simulink model "torch_arm_telem"  (R2024a)
settings: Solver=FixedStepAuto  StartTime=0.0  StopTime=50  FixedStep=framePeriod_s  RelTol=1e-3
undefined symbols (not defined in the file): Aircraft, DiscIntNeverNeededParam, framePeriod_s, frameRate_hz, magnitude
libraries: simulink x42, slpidlib x13, dspmathops x1, simulink_extras x1
(part 2 of 4)

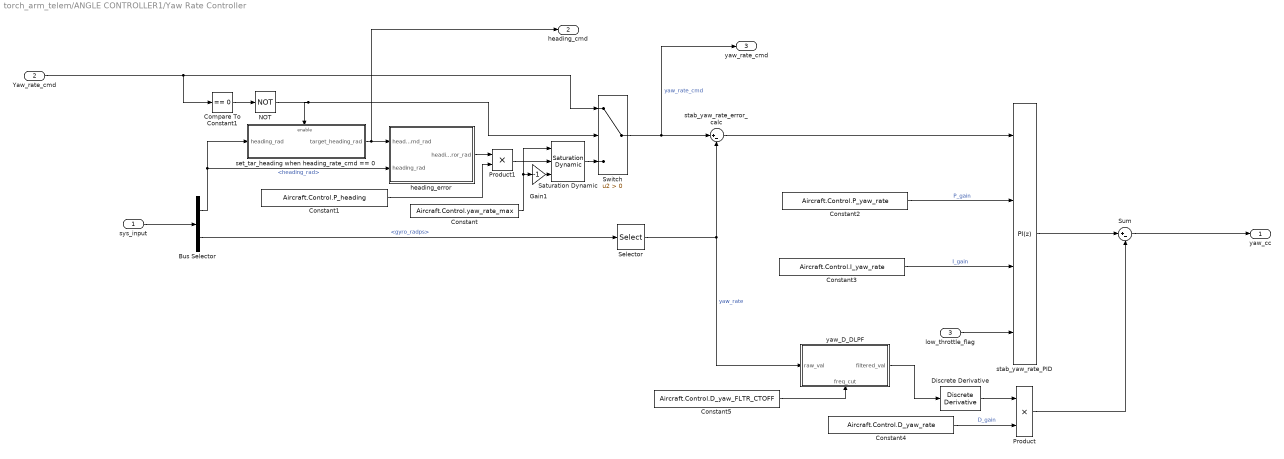
== system torch_arm_telem/ANGLE CONTROLLER1/Yaw Rate Controller ==
  sys_input : Inport
  Yaw_rate_cmd : Inport  Port=2
  low_throttle_flag : Inport  Port=3
  Bus Selector : BusSelector  OutputSignals=StateEstData.bfs_ins.heading_rad,StateEstData.bfs_ins.gyro_radps
  Compare To Constant1 : simulink/Logic and Bit Operations/Compare To Constant  relop===  const=0  OutDataTypeStr=boolean
  Constant : Constant  Value=Aircraft.Control.yaw_rate_max
  Constant1 : Constant  Value=Aircraft.Control.P_heading  OutDataTypeStr=single
  Constant2 : Constant  Value=Aircraft.Control.P_yaw_rate  OutDataTypeStr=single
  Constant3 : Constant  Value=Aircraft.Control.I_yaw_rate  OutDataTypeStr=single
  Constant4 : Constant  Value=Aircraft.Control.D_yaw_rate  OutDataTypeStr=single
  Constant5 : Constant  Value=Aircraft.Control.D_yaw_FLTR_CTOFF  OutDataTypeStr=single
  Discrete Derivative : simulink/Quick Insert/Discrete/Discrete Derivative  gainval=1.0  ICPrevScaledInput=0.0  OutMin=[]  OutMax=[]  OutDataType=fixdt(1, 16)  OutScaling=2^-10  DoSatur=off
  Gain1 : Gain  Gain=-1
  NOT : Logic  Operator=NOT  IconShape=distinctive  AllPortsSameDT=off  OutDataTypeStr=boolean
  Product : Product
  Product1 : Product
  Saturation Dynamic : simulink/Discontinuities/Saturation Dynamic  OutMin=[]  OutMax=[]  OutDataTypeStr=Inherit: Same as second input  OutDataType=fixdt(1, 16)  OutScaling=2^-10  DoSatur=off
  Selector : Selector  InputPortWidth=3  IndexOptions=Index vector (dialog)  Indices=3  OutputSizes=1
  Sum : Sum  Inputs=|+-
  Switch : Switch  Criteria=u2 > Threshold  SaturateOnIntegerOverflow=off  InputSameDT=off
  heading_error : Subsystem
  set_tar_heading when heading_rate_cmd == 0 : Subsystem  TreatAsAtomicUnit=on
  stab_yaw_rate_PID : slpidlib/PID Controller  Controller=PI  Form=Parallel  TimeDomain=Discrete-time  UseExternalTs=off  SampleTime=framePeriod_s  IntegratorMethod=Forward Euler  FilterMethod=Forward Euler  ControllerParametersSource=external  P=1.85  I=0.01  UseKiTs=off  D=0  UseExternalDerivativeSource=off  N=100  UseFilter=off  TunerSelectOption=Transfer Function Based (PID Tuner App)  InitialConditionSource=internal  InitialConditionForIntegrator=0  InitialConditionForFilter=0  DifferentiatorICPrevScaledInput=0  ExternalReset=either  TrackingMode=off  Kt=1  LimitOutput=on  SatLimitsSource=internal  UpperSaturationLimit=1  LowerSaturationLimit=-1  LinearizeAsGain=off  AntiWindupMode=clamping  Kb=1  LimitIntegrator=off  UpperIntegratorSaturationLimit=inf  LowerIntegratorSaturationLimit=-inf  POutMin=[]  POutMax=[]  IOutMin=[]  IOutMax=[]  DOutMin=[]  DOutMax=[]  NOutMin=[]  NOutMax=[]  SumOutMin=[]  SumOutMax=[]  SaturationOutMin=[]  SaturationOutMax=[]  PParamMin=[]  PParamMax=[]  IParamMin=[]  IParamMax=[]  DParamMin=[]  DParamMax=[]  NParamMin=[]  NParamMax=[]  KbParamMin=[]  KbParamMax=[]  KtParamMin=[]  KtParamMax=[]  KbOutMin=[]  KbOutMax=[]  KtOutMin=[]  KtOutMax=[]  IntegratorOutMin=[]  IntegratorOutMax=[]  FilterOutMin=[]  FilterOutMax=[]  SumI1OutMin=[]  SumI1OutMax=[]  SumI2OutMin=[]  SumI2OutMax=[]  SumI3OutMin=[]  SumI3OutMax=[]  SumI4OutMin=[]  SumI4OutMax=[]  SumDOutMin=[]  SumDOutMax=[]  DifferentiatorOutMin=[]  DifferentiatorOutMax=[]  FilterDiffOutCoefMin=[]  FilterDiffOutCoefMax=[]  ReciprocalOutMin=[]  ReciprocalOutMax=[]  SumDenOutMin=[]  SumDenOutMax=[]  SumNumOutMin=[]  SumNumOutMax=[]  DivideOutMin=[]  DivideOutMax=[]  UdiffTsProdOutMin=[]  UdiffTsProdOutMax=[]  NTsProdOutMin=[]  NTsProdOutMax=[]  UintegralTsProdOutMin=[]  UintegralTsProdOutMax=[]  UngainTsProdOutMin=[]  UngainTsProdOutMax=[]  ClampingZeroOutDataTypeStr=Inherit: Inherit via back propagation  ClampingZeroOutMin=[]  ClampingZeroOutMax=[]  FilterDenConstantOutDataTypeStr=Inherit: Inherit via back propagation  FilterDenConstantOutMin=[]  FilterDenConstantOutMax=[]  PCopyOutDataTypeStr=Inherit: Inherit via back propagation  PCopyOutMin=[]  PCopyOutMax=[]  NCopyOutDataTypeStr=Inherit: Inherit via back propagation  NCopyOutMin=[]  NCopyOutMax=[]  IntegratorContinuousStateAttributes=''  IntegratorStateMustResolveToSignalObject=off  IntegratorRTWStateStorageClass=Auto  FilterContinuousStateAttributes=''  FilterStateMustResolveToSignalObject=off  FilterRTWStateStorageClass=Auto  ParallelPVariant=ExternalParameters  IdealPVariant=Disabled  IVariant=ExternalParameters  DVariant=Disabled  IntegratorVariant=Discrete  SatVariant=Enabled  AWVariant=DiscClampingParallel  PCopyVariant=Disabled  TRVariant=Disabled  FdbkBlocksVariant=Forward  IdealPFdbkVariant=Disabled  SatFdbkVariant=Disabled  DerivativeFilterVariant=Disabled  NVariant=Disabled  NCopyVariant=Disabled_SignalSpec  FilterICVariant=Disabled  IntegratorICVariant=InternalICs  ExternalResetVariant=ExternalReset  TRSumVariant=Passthrough  SumFdbkVariant=Disabled  SumVariant=Sum_PI  TsampFilterVariant=InternalTs  TsampNgainVariant=Passthrough  TsampIntegralVariant=Disabled_SignalSpec  ExternalSaturationOutDataTypeStr=Inherit: Same as second input  DerivativeSourceVariant=Disabled
  stab_yaw_rate_error_calc : Sum  Inputs=|+-
  yaw_D_DLPF : Subsystem
      settings: PortSchema="{\"entries\":[{\"content\":{\"sides\":[{\"content\":{\"connectorIds\":[\"In1\"]},\"type\":\"ConnectorPlacement.EquallySpacedRectSide\",\"uuid\":\"20236834-aeb3-4c5b-bb2e-f84447e752b5\"},{\"content\":{\"connectorIds\":[\"Out1\"],\"side\":\"RIGHT\"},\"type\":\"ConnectorPlacement.EquallySpacedRectSide\",\"uuid\":\"d668f9a1-a3df-4207-8bf1-99fb838e59b2\"},{\"content\":{\"connectorIds\":[],\"side\":\"TOP\"},\"type\":\"ConnectorPlacement.EquallySpacedRectSide\",\"uuid\":\"66cceb06-f4bc-4278-b965-2427292e46df\"},{\"content\":{\"connectorIds\":[\"In2\"],\"side\":\"BOTTOM\"},\"type\":\"ConnectorPlacement.EquallySpacedRectSide\",\"uuid\":\"8fdaac6a-cb03-4bd4-87bb-7bafd10bc297\"}]},\"type\":\"ConnectorPlacement.EquallySpacedConnector\",\"uuid\":\"3dc29a9a-e794-478d-b7df-452e6c2d3f66\"}],\"packageUris\":[\"http://schema.mathworks.com/mf0/Connector/R2020b\"],\"version\":\"1.0\"}"
  yaw_cc : Outport
  heading_cmd : Outport  Port=2
  yaw_rate_cmd : Outport  Port=3
  wires:
  sys_input/1 -> Bus Selector/1
  Bus Selector/2 -> Selector/1  "<gyro_radps>"
  stab_yaw_rate_PID/1 -> Sum/1
  Sum/1 -> yaw_cc/1
  Product/1 -> Sum/2
  Discrete Derivative/1 -> Product/1
  Constant2/1 -> stab_yaw_rate_PID/2  "P_gain"
  Constant3/1 -> stab_yaw_rate_PID/3  "I_gain"
  Constant4/1 -> Product/2  "D_gain"
  Selector/1 -> stab_yaw_rate_error_calc/2, yaw_D_DLPF/1(raw_val)  "yaw_rate"
  low_throttle_flag/1 -> stab_yaw_rate_PID/4
  Compare To Constant1/1 -> NOT/1
  Bus Selector/1 -> set_tar_heading when heading_rate_cmd == 0/1(heading_rad), heading_error/2(heading_rad)  "<heading_rad>"
  Switch/1 -> yaw_rate_cmd/1, stab_yaw_rate_error_calc/1  "yaw_rate_cmd"
  Yaw_rate_cmd/1 -> Switch/1, Compare To Constant1/1
  heading_error/1(heading_error_rad) -> Product1/1
  Constant1/1 -> Product1/2
  NOT/1 -> Switch/2, set_tar_heading when heading_rate_cmd == 0/Enable
  set_tar_heading when heading_rate_cmd == 0/1(target_heading_rad) -> heading_cmd/1, heading_error/1(heading_cmd_rad)
  Product1/1 -> Saturation Dynamic/2
  Saturation Dynamic/1 -> Switch/3
  Gain1/1 -> Saturation Dynamic/3
  Constant/1 -> Saturation Dynamic/1, Gain1/1
  Constant5/1 -> yaw_D_DLPF/2(freq_cut)
  yaw_D_DLPF/1(filtered_val) -> Discrete Derivative/1
  stab_yaw_rate_error_calc/1 -> stab_yaw_rate_PID/1

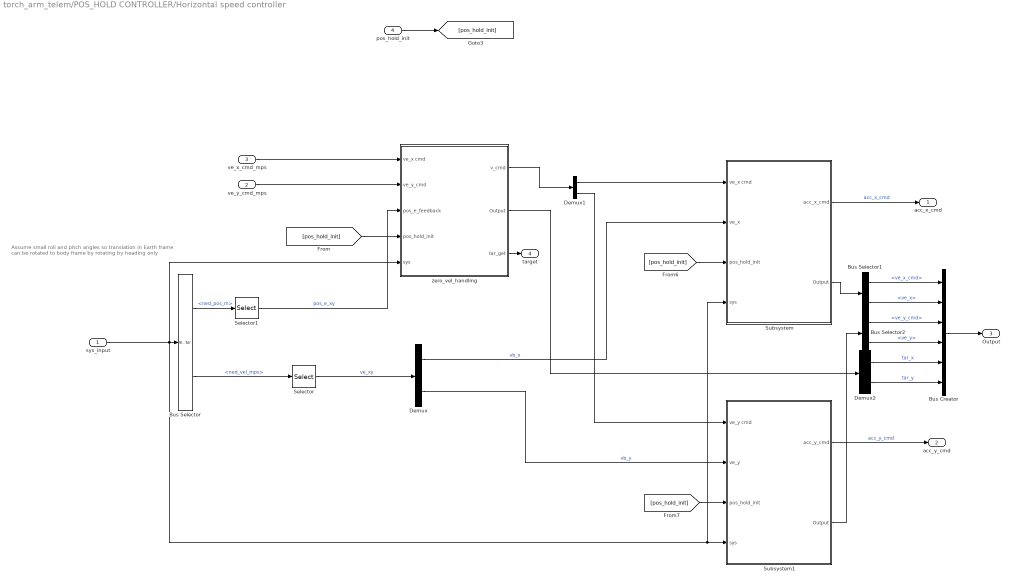
== system torch_arm_telem/POS_HOLD CONTROLLER/Horizontal speed controller ==
  note: Assume small roll and pitch angles so translation in Earth frame can be rotated to body frame by rotating by heading only
  sys_input : Inport
  ve_y_cmd_mps : Inport  Port=2
  ve_x_cmd_mps : Inport  Port=3
  pos_hold_init : Inport  Port=4
  Bus Creator : BusCreator  Inputs=6
  Bus Selector : BusSelector  OutputSignals=StateEstData.aux_ins.ned_pos_m,StateEstData.bfs_ins.ned_vel_mps
  Bus Selector1 : BusSelector  OutputSignals=ve_x_cmd,ve_x
  Bus Selector2 : BusSelector  OutputSignals=ve_y_cmd,ve_y
  Demux : Demux  Outputs=2
  Demux1 : Demux  Outputs=2
  Demux2 : Demux  Outputs=2
  Selector : Selector  InputPortWidth=3  IndexOptions=Index vector (dialog)  Indices=[1 2]  OutputSizes=1
  Selector1 : Selector  InputPortWidth=3  IndexOptions=Index vector (dialog)  Indices=[1 2]  OutputSizes=1
  Subsystem : Subsystem
  Subsystem1 : Subsystem
  zero_vel_handling : Subsystem
  acc_x_cmd : Outport
  acc_y_cmd : Outport  Port=2
  Output : Outport  Port=3
  target : Outport  Port=4
  wires:
  Subsystem1/1(acc_y_cmd) -> acc_y_cmd/1  "acc_y_cmd"
  Subsystem/1(acc_x_cmd) -> acc_x_cmd/1  "acc_x_cmd"
  sys_input/1 -> Bus Selector/1, Subsystem/4(sys), Subsystem1/4(sys), zero_vel_handling/5(sys)
  Bus Selector/2 -> Selector/1  "<ned_vel_mps>"
  Demux/1 -> Subsystem/2(ve_x)  "vb_x"
  pos_hold_init/1 -> [pos_hold_init]
  [pos_hold_init] -> Subsystem/3(pos_hold_init)
  [pos_hold_init] -> Subsystem1/3(pos_hold_init)
  Subsystem/2(Output) -> Bus Selector1/1
  Subsystem1/2(Output) -> Bus Selector2/1
  Bus Selector1/1 -> Bus Creator/1  "<ve_x_cmd>"
  Bus Selector1/2 -> Bus Creator/2  "<ve_x>"
  Bus Selector2/1 -> Bus Creator/3  "<ve_y_cmd>"
  Bus Selector2/2 -> Bus Creator/4  "<ve_y>"
  Bus Creator/1 -> Output/1
  Bus Selector/1 -> Selector1/1  "<ned_pos_m>"
  Demux/2 -> Subsystem1/2(ve_y)  "vb_y"
  ve_x_cmd_mps/1 -> zero_vel_handling/1(ve_x cmd)
  ve_y_cmd_mps/1 -> zero_vel_handling/2(ve_y_cmd)
  Selector1/1 -> zero_vel_handling/3(pos_e_feedback)  "pos_e_xy"
  [pos_hold_init] -> zero_vel_handling/4(pos_hold_init)
  zero_vel_handling/1(v_cmd) -> Demux1/1
  Demux1/1 -> Subsystem/1(ve_x cmd)
  Demux1/2 -> Subsystem1/1(ve_y cmd)
  zero_vel_handling/2(Output) -> Demux2/1
  Demux2/1 -> Bus Creator/5  "tar_x"
  Demux2/2 -> Bus Creator/6  "tar_y"
  Selector/1 -> Demux/1  "ve_xy"
  zero_vel_handling/3(tar_get) -> target/1

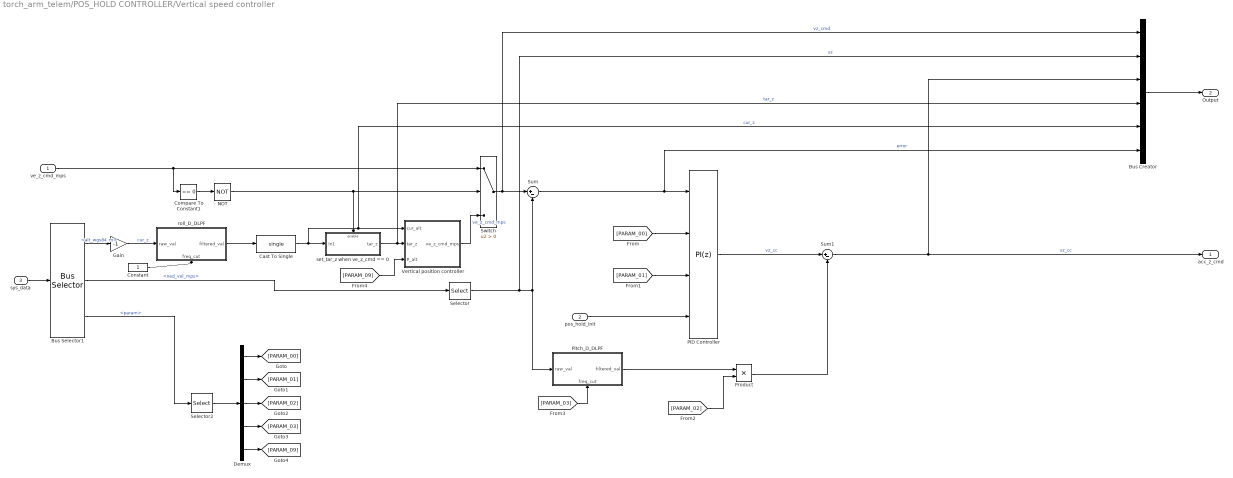
== system torch_arm_telem/POS_HOLD CONTROLLER/Vertical speed controller ==
  ve_z_cmd_mps : Inport
  pos_hold_init : Inport  Port=2
  sys_data : Inport  Port=3
  Bus Creator : BusCreator  Inputs=6
  Bus Selector1 : BusSelector  OutputSignals=Sensor Data.ext_gnss1.alt_wgs84_m,StateEstData.bfs_ins.ned_vel_mps,Telemetry Data.param
  Cast To Single : DataTypeConversion  OutDataTypeStr=single  SaturateOnIntegerOverflow=off  RndMeth=Floor
  Compare To Constant1 : simulink/Logic and Bit Operations/Compare To Constant  relop===  const=0  OutDataTypeStr=boolean
  Constant : Constant  OutDataTypeStr=single
  Demux : Demux  Outputs=5
  Gain : Gain  Gain=-1
  NOT : Logic  Operator=NOT  IconShape=distinctive  AllPortsSameDT=off  OutDataTypeStr=boolean
  PID Controller : slpidlib/PID Controller  Controller=PI  Form=Parallel  TimeDomain=Discrete-time  UseExternalTs=off  SampleTime=framePeriod_s  IntegratorMethod=Forward Euler  FilterMethod=Forward Euler  ControllerParametersSource=external  P=0  I=0  UseKiTs=off  D=0  UseExternalDerivativeSource=off  N=100  UseFilter=off  TunerSelectOption=Frequency Response Based  InitialConditionSource=internal  InitialConditionForIntegrator=0  InitialConditionForFilter=0  DifferentiatorICPrevScaledInput=0  ExternalReset=either  TrackingMode=off  Kt=1  LimitOutput=on  SatLimitsSource=internal  UpperSaturationLimit=1  LowerSaturationLimit=-1  LinearizeAsGain=on  AntiWindupMode=clamping  Kb=1  LimitIntegrator=off  UpperIntegratorSaturationLimit=inf  LowerIntegratorSaturationLimit=-inf  POutMin=[]  POutMax=[]  IOutMin=[]  IOutMax=[]  DOutMin=[]  DOutMax=[]  NOutMin=[]  NOutMax=[]  SumOutMin=[]  SumOutMax=[]  SaturationOutMin=[]  SaturationOutMax=[]  PParamMin=[]  PParamMax=[]  IParamMin=[]  IParamMax=[]  DParamMin=[]  DParamMax=[]  NParamMin=[]  NParamMax=[]  KbParamMin=[]  KbParamMax=[]  KtParamMin=[]  KtParamMax=[]  KbOutMin=[]  KbOutMax=[]  KtOutMin=[]  KtOutMax=[]  IntegratorOutMin=[]  IntegratorOutMax=[]  FilterOutMin=[]  FilterOutMax=[]  SumI1OutMin=[]  SumI1OutMax=[]  SumI2OutMin=[]  SumI2OutMax=[]  SumI3OutMin=[]  SumI3OutMax=[]  SumI4OutMin=[]  SumI4OutMax=[]  SumDOutMin=[]  SumDOutMax=[]  DifferentiatorOutMin=[]  DifferentiatorOutMax=[]  FilterDiffOutCoefMin=[]  FilterDiffOutCoefMax=[]  ReciprocalOutMin=[]  ReciprocalOutMax=[]  SumDenOutMin=[]  SumDenOutMax=[]  SumNumOutMin=[]  SumNumOutMax=[]  DivideOutMin=[]  DivideOutMax=[]  UdiffTsProdOutMin=[]  UdiffTsProdOutMax=[]  NTsProdOutMin=[]  NTsProdOutMax=[]  UintegralTsProdOutMin=[]  UintegralTsProdOutMax=[]  UngainTsProdOutMin=[]  UngainTsProdOutMax=[]  ClampingZeroOutDataTypeStr=Inherit: Inherit via back propagation  ClampingZeroOutMin=[]  ClampingZeroOutMax=[]  FilterDenConstantOutDataTypeStr=Inherit: Inherit via back propagation  FilterDenConstantOutMin=[]  FilterDenConstantOutMax=[]  PCopyOutDataTypeStr=Inherit: Inherit via back propagation  PCopyOutMin=[]  PCopyOutMax=[]  NCopyOutDataTypeStr=Inherit: Inherit via back propagation  NCopyOutMin=[]  NCopyOutMax=[]  IntegratorContinuousStateAttributes=''  IntegratorStateMustResolveToSignalObject=off  IntegratorRTWStateStorageClass=Auto  FilterContinuousStateAttributes=''  FilterStateMustResolveToSignalObject=off  FilterRTWStateStorageClass=Auto  ParallelPVariant=ExternalParameters  IdealPVariant=Disabled  IVariant=ExternalParameters  DVariant=Disabled  IntegratorVariant=Discrete  SatVariant=Enabled  AWVariant=DiscClampingParallel  PCopyVariant=Disabled  TRVariant=Disabled  FdbkBlocksVariant=Forward  IdealPFdbkVariant=Disabled  SatFdbkVariant=Disabled  DerivativeFilterVariant=Disabled  NVariant=Disabled  NCopyVariant=Disabled_SignalSpec  FilterICVariant=Disabled  IntegratorICVariant=InternalICs  ExternalResetVariant=ExternalReset  TRSumVariant=Passthrough  SumFdbkVariant=Disabled  SumVariant=Sum_PI  TsampFilterVariant=InternalTs  TsampNgainVariant=Passthrough  TsampIntegralVariant=Disabled_SignalSpec  ExternalSaturationOutDataTypeStr=Inherit: Same as second input  DerivativeSourceVariant=Disabled
  Pitch_D_DLPF : Subsystem
      settings: PortSchema="{\"entries\":[{\"content\":{\"sides\":[{\"content\":{\"connectorIds\":[\"In1\"]},\"type\":\"ConnectorPlacement.EquallySpacedRectSide\",\"uuid\":\"20236834-aeb3-4c5b-bb2e-f84447e752b5\"},{\"content\":{\"connectorIds\":[\"Out1\"],\"side\":\"RIGHT\"},\"type\":\"ConnectorPlacement.EquallySpacedRectSide\",\"uuid\":\"d668f9a1-a3df-4207-8bf1-99fb838e59b2\"},{\"content\":{\"connectorIds\":[],\"side\":\"TOP\"},\"type\":\"ConnectorPlacement.EquallySpacedRectSide\",\"uuid\":\"66cceb06-f4bc-4278-b965-2427292e46df\"},{\"content\":{\"connectorIds\":[\"In2\"],\"side\":\"BOTTOM\"},\"type\":\"ConnectorPlacement.EquallySpacedRectSide\",\"uuid\":\"7d08bc25-8e2d-44c6-8f94-b04e75c70268\"}]},\"type\":\"ConnectorPlacement.EquallySpacedConnector\",\"uuid\":\"3dc29a9a-e794-478d-b7df-452e6c2d3f66\"}],\"packageUris\":[\"http://schema.mathworks.com/mf0/Connector/R2020b\"],\"version\":\"1.0\"}"
  Product : Product
  Selector : Selector  InputPortWidth=3  IndexOptions=Index vector (dialog)  Indices=[3]  OutputSizes=1
  Selector2 : Selector  IndexMode=Zero-based  InputPortWidth=24  IndexOptions=Index vector (dialog)  Indices=[0 1 2 3 9]  OutputSizes=1
  Sum : Sum  Inputs=|+-
  Sum1 : Sum  Inputs=|+-
  Switch : Switch  Criteria=u2 > Threshold  SaturateOnIntegerOverflow=off  InputSameDT=off
  Vertical position controller : Subsystem
  roll_D_DLPF : Subsystem
      settings: PortSchema="{\"entries\":[{\"content\":{\"sides\":[{\"content\":{\"connectorIds\":[\"In1\"]},\"type\":\"ConnectorPlacement.EquallySpacedRectSide\",\"uuid\":\"20236834-aeb3-4c5b-bb2e-f84447e752b5\"},{\"content\":{\"connectorIds\":[\"Out1\"],\"side\":\"RIGHT\"},\"type\":\"ConnectorPlacement.EquallySpacedRectSide\",\"uuid\":\"d668f9a1-a3df-4207-8bf1-99fb838e59b2\"},{\"content\":{\"connectorIds\":[],\"side\":\"TOP\"},\"type\":\"ConnectorPlacement.EquallySpacedRectSide\",\"uuid\":\"66cceb06-f4bc-4278-b965-2427292e46df\"},{\"content\":{\"connectorIds\":[\"In2\"],\"side\":\"BOTTOM\"},\"type\":\"ConnectorPlacement.EquallySpacedRectSide\",\"uuid\":\"8fdaac6a-cb03-4bd4-87bb-7bafd10bc297\"}]},\"type\":\"ConnectorPlacement.EquallySpacedConnector\",\"uuid\":\"3dc29a9a-e794-478d-b7df-452e6c2d3f66\"}],\"packageUris\":[\"http://schema.mathworks.com/mf0/Connector/R2020b\"],\"version\":\"1.0\"}"
  set_tar_z when ve_z_cmd == 0 : Subsystem  TreatAsAtomicUnit=on
  acc_z_cmd : Outport
  Output : Outport  Port=2
  wires:
  [PARAM_00] -> PID Controller/2
  Bus Selector1/2 -> Selector/1  "<ned_vel_mps>"
  sys_data/1 -> Bus Selector1/1
  Pitch_D_DLPF/1(filtered_val) -> Product/1
  Selector/1 -> Bus Creator/2, Sum/2, Pitch_D_DLPF/1(raw_val)  "vz"
  [PARAM_02] -> Product/2
  Product/1 -> Sum1/2
  ve_z_cmd_mps/1 -> Compare To Constant1/1, Switch/1
  Compare To Constant1/1 -> NOT/1
  Switch/1 -> Bus Creator/1, Sum/1  "vz_cmd"
  set_tar_z when ve_z_cmd == 0/1(tar_z) -> Bus Creator/4, Vertical position controller/2(tar_z)  "tar_z"
  pos_hold_init/1 -> PID Controller/4
  [PARAM_03] -> Pitch_D_DLPF/2(freq_cut)
  [PARAM_09] -> Vertical position controller/3(P_alt)
  Bus Creator/1 -> Output/1
  Cast To Single/1 -> Bus Creator/5, Vertical position controller/1(cur_alt), set_tar_z when ve_z_cmd == 0/1(In1)  "cur_z"
  Sum/1 -> Bus Creator/6, PID Controller/1  "error"
  Sum1/1 -> acc_z_cmd/1, Bus Creator/3  "vz_cc"
  PID Controller/1 -> Sum1/1  "vz_cc"
  Bus Selector1/3 -> Selector2/1  "<param>"
  Selector2/1 -> Demux/1
  Demux/1 -> [PARAM_00]
  Demux/2 -> [PARAM_01]
  Demux/3 -> [PARAM_02]
  Demux/4 -> [PARAM_03]
  [PARAM_01] -> PID Controller/3
  Vertical position controller/1(ve_z_cmd_mps) -> Switch/3  "ve_z_cmd_mps"
  Demux/5 -> [PARAM_09]
  NOT/1 -> Switch/2, set_tar_z when ve_z_cmd == 0/Enable
  Bus Selector1/1 -> Gain/1  "<alt_wgs84_m>"
  Gain/1 -> roll_D_DLPF/1(raw_val)  "cur_z"
  roll_D_DLPF/1(filtered_val) -> Cast To Single/1
  Constant/1 -> roll_D_DLPF/2(freq_cut)

== system torch_arm_telem/POS_HOLD_input_conversion/body_to_inertial conversion ==
  vb_xy : Inport
  heading_rad : Inport  Port=2
  2D rotation from NED_xy to body_xy : Subsystem
  Demux : Demux  Outputs=2
  Product : Product  Multiplication=Matrix(*)
  Transpose : Math  Operator=transpose
  ve_x : Outport
  ve_y : Outport  Port=2
  wires:
  Demux/1 -> ve_x/1  "ve_x"
  Product/1 -> Demux/1  "ve_xy"
  heading_rad/1 -> 2D rotation from NED_xy to body_xy/1(<heading_rad>)
  vb_xy/1 -> Product/2
  2D rotation from NED_xy to body_xy/1(2D_rot) -> Transpose/1
  Demux/2 -> ve_y/1  "ve_y"
  Transpose/1 -> Product/1

== system torch_arm_telem/POS_HOLD_input_conversion/pitch_norm_deadband ==
  raw_sbus_in : Inport
  deadband : Inport  Port=2
  Constant : Constant  Value=0  OutDataTypeStr=single
  Constant1 : Constant  Value=Aircraft.Control.v_z_max  OutDataTypeStr=single
  Constant2 : Constant  Value=-Aircraft.Control.v_z_max  OutDataTypeStr=single
  Constant3 : Constant  OutDataTypeStr=single
  remap_with_deadband : MATLAB Function  TreatAsAtomicUnit=on
  normalized_out : Outport
  wires:
  deadband/1 -> remap_with_deadband/6(deadband)
  Constant2/1 -> remap_with_deadband/5(out_max)
  Constant1/1 -> remap_with_deadband/4(out_min)
  Constant3/1 -> remap_with_deadband/3(in_max)
  Constant/1 -> remap_with_deadband/2(in_min)
  remap_with_deadband/1(norm_out) -> normalized_out/1
  raw_sbus_in/1 -> remap_with_deadband/1(raw_in)

== system torch_arm_telem/Stab_input_conversion/remap from min_spin to max ==
  raw_in : Inport
  Constant4 : Constant  Value=0  OutDataTypeStr=single
  Constant5 : Constant  Value=Aircraft.Control.motor_spin_min  OutDataTypeStr=single
  Constant6 : Constant  OutDataTypeStr=single
  Constant7 : Constant  OutDataTypeStr=single
  remap1 : MATLAB Function  TreatAsAtomicUnit=on
  norm_out : Outport
  wires:
  Constant6/1 -> remap1/5(out_max)
  Constant5/1 -> remap1/4(out_min)
  remap1/1(norm_out) -> norm_out/1
  Constant4/1 -> remap1/2(in_min)
  Constant7/1 -> remap1/3(in_max)
  raw_in/1 -> remap1/1(raw_in)

== system torch_arm_telem/WAYPOINT CONTROLLER/WP_NAV ==
  Cmd : Inport
  Sys_input : Inport  Port=2
  cur_target_pos_m : Inport  Port=3
  prev_pos_m : Inport  Port=4
  max_v_hor_mps : Inport  Port=5
  max_v_z_mps : Inport  Port=6
  Enable : EnablePort
  Bus Creator4 : BusCreator  Inputs=4
  Bus Selector : BusSelector  OutputSignals=yaw_rate_cmd_radps
  Horizontal position controller : Subsystem
  Subsystem : Subsystem
  Vertical position controller : Subsystem  Commented=on
  heading_controller : Subsystem  Commented=on
  Command out : Outport
  nav_data : Outport  Port=2
  wires:
  Bus Creator4/1 -> Command out/1
  Horizontal position controller/1(ve_x_cmd_mps) -> Bus Creator4/2  "ve_x_cmd_mps"
  Horizontal position controller/2(ve_y_cmd_mps) -> Bus Creator4/3  "ve_y_cmd_mps"
  Sys_input/1 -> Horizontal position controller/1(Sys_input), Subsystem/1(Sys_input)
  cur_target_pos_m/1 -> Subsystem/2(tar_pos), Horizontal position controller/2(cur_target_pos_m)
  Cmd/1 -> Bus Selector/1
  Bus Selector/1 -> Bus Creator4/4  "<yaw_rate_cmd_radps>"
  prev_pos_m/1 -> Horizontal position controller/3(prev_pos_m)
  max_v_hor_mps/1 -> Horizontal position controller/4(max_v_hor_mps)
  Subsystem/1(ve_z_cmd_mps) -> Bus Creator4/1  "ve_z_cmd_mps"
  max_v_z_mps/1 -> Subsystem/3(max_v_z_mps)
  Horizontal position controller/3(nav_data) -> nav_data/1

== system torch_arm_telem/WAYPOINT CONTROLLER/capture rising edge ==
  <current_waypoint> : Inport
  Detect Change1 : simulink/Logic and Bit Operations/Detect Change  vinit=-1  OutDataTypeStr=boolean
  Detect Rise Positive : simulink/Logic and Bit Operations/Detect Rise Positive  Commented=through  vinit=0  OutDataTypeStr=boolean
  enable : Outport
  wires:
  <current_waypoint>/1 -> Detect Change1/1
  Detect Rise Positive/1 -> enable/1
  Detect Change1/1 -> Detect Rise Positive/1

== system torch_arm_telem/WAYPOINT CONTROLLER/determine target ==
  sys_input : Inport
  Enable : EnablePort  PropagateVarSize=During execution
  Bus Selector : BusSelector  OutputSignals=Telemetry Data.flight_plan,Telemetry Data.current_waypoint,StateEstData.aux_ins.home_lat_rad,StateEstData.aux_ins.home_lon_rad,StateEstData.aux_ins.home_alt_wgs84_m,StateEstData.aux_ins.ned_pos_m
  Bus Selector1 : BusSelector  OutputSignals=x,y,z,frame
  Cast To Single1 : DataTypeConversion  OutDataTypeStr=single  SaturateOnIntegerOverflow=off  RndMeth=Floor
  Cast To Single2 : DataTypeConversion  OutDataTypeStr=single  SaturateOnIntegerOverflow=off  RndMeth=Floor
  Constant : Constant  OutDataTypeStr=int16
  Constant1 : Constant  Value=4  OutDataTypeStr=uint8
  Constant2 : Constant  Value=Aircraft.Control.nav_speed  OutDataTypeStr=single
  Constant3 : Constant  Value=Aircraft.Control.v_z_max  OutDataTypeStr=single
  Gain : Gain  Gain=0.0000001  OutDataTypeStr=double
  Gain1 : Gain  Gain=0.0000001  OutDataTypeStr=double
  Selector1 : Selector  IndexMode=Zero-based  InputPortWidth=500  IndexOptions=Index vector (port)  Indices=[1 3]  OutputSizes=1
  Sum : Sum  Inputs=|++
  Unit Delay : UnitDelay  InitialCondition=[0 0 0]  SampleTime=-1  HasFrameUpgradeWarning=on
  determine max speeds : MATLAB Function  TreatAsAtomicUnit=on
  determine_current_tar_pos : MATLAB Function  TreatAsAtomicUnit=on
  cur_target_pos_m : Outport
  prev_pos_m : Outport  Port=2
  max_v_xy_mps : Outport  Port=3
  max_v_z_mps : Outport  Port=4
  wires:
  sys_input/1 -> Bus Selector/1
  Selector1/1 -> Bus Selector1/1
  Bus Selector1/3 -> determine_current_tar_pos/3(fp_z)  "<z>"
  Bus Selector1/2 -> Gain1/1  "<y>"
  Bus Selector1/1 -> Gain/1  "<x>"
  Bus Selector/1 -> Selector1/1  "<flight_plan>"
  Bus Selector/3 -> determine_current_tar_pos/5(home_lat_rad)  "<home_lat_rad>"
  Bus Selector/4 -> determine_current_tar_pos/6(home_lon_rad)  "<home_lon_rad>"
  Bus Selector/5 -> determine_current_tar_pos/7(home_alt)  "<home_alt_wgs84_m>"
  Gain/1 -> Cast To Single1/1
  Gain1/1 -> Cast To Single2/1
  Bus Selector/2 -> Sum/1  "<current_waypoint>"
  Sum/1 -> Selector1/2
  Constant/1 -> Sum/2
  Constant1/1 -> determine_current_tar_pos/4(wp_frame)
  Unit Delay/1 -> prev_pos_m/1
  determine_current_tar_pos/1(cur_target_pos) -> determine max speeds/1(cur_tar_pos), cur_target_pos_m/1, Unit Delay/1
  Cast To Single1/1 -> determine_current_tar_pos/1(fp_x)
  Cast To Single2/1 -> determine_current_tar_pos/2(fp_y)
  Bus Selector/6 -> determine max speeds/2(cur_pos)  "<ned_pos_m>"
  Constant2/1 -> determine max speeds/3(max_hor_spd)
  Constant3/1 -> determine max speeds/4(max_ver_spd)
  determine max speeds/1(max_v_z_mps) -> max_v_z_mps/1
  determine max speeds/2(max_v_xy_mps) -> max_v_xy_mps/1

== system torch_arm_telem/WAYPOINT CONTROLLER/wp_completion_check ==
  note: Output wp_reached cmd only when distance between current pos and target pos is less than wp_radius.
  target_pos : Inport
  Sys_input : Inport  Port=2
  Bus Selector : BusSelector  OutputSignals=StateEstData.aux_ins.ned_pos_m
  Constant : Constant  Value=Aircraft.Control.wp_radius  OutDataTypeStr=single
  check_wp_reached : MATLAB Function  TreatAsAtomicUnit=on
  wp_reached : Outport
  wires:
  Sys_input/1 -> Bus Selector/1
  Bus Selector/1 -> check_wp_reached/2(ned_pos)  "<ned_pos_m>"
  check_wp_reached/1(reached) -> wp_reached/1
  target_pos/1 -> check_wp_reached/1(target_pos)
  Constant/1 -> check_wp_reached/3(Aircraft_Control_wp_radius)

== system torch_arm_telem/WAYPOINT CONTROLLER CMD/Throttle Mapper ==
  Throttle : Inport
  Compare To Constant : simulink/Logic and Bit Operations/Compare To Constant  relop=<  const=0  OutDataTypeStr=boolean
  Compare To Constant1 : simulink/Logic and Bit Operations/Compare To Constant  relop=>=  const=0  OutDataTypeStr=boolean
  Constant : Constant  Value=Aircraft.Control.v_z_down_max  OutDataTypeStr=single
  Constant1 : Constant  Value=Aircraft.Control.v_z_up_max  OutDataTypeStr=single
  Double : Constant  Value=2  OutDataTypeStr=single
  Gain : Gain  Gain=-1
  Normalize at Zero : Constant  Value=0.5  OutDataTypeStr=single
  Product : Product  Inputs=3
  Product1 : Product  Inputs=3
  Sum : Sum  Inputs=|+-
  Sum1 : Sum
  v_z_cmd (-1 to 1) : Product
  Relative Velocity : Outport
  wires:
  Throttle/1 -> Sum/1
  Normalize at Zero/1 -> Sum/2
  Double/1 -> v_z_cmd (-1 to 1)/2
  Sum/1 -> v_z_cmd (-1 to 1)/1
  Sum1/1 -> Gain/1
  v_z_cmd (-1 to 1)/1 -> Product1/2, Compare To Constant1/1, Compare To Constant/1, Product/3
  Constant1/1 -> Product1/3
  Compare To Constant1/1 -> Product1/1
  Product/1 -> Sum1/1
  Product1/1 -> Sum1/2
  Constant/1 -> Product/1
  Compare To Constant/1 -> Product/2
  Gain/1 -> Relative Velocity/1

== system torch_arm_telem/WAYPOINT CONTROLLER CMD/pitch_norm_deadband ==
  raw_sbus_in : Inport
  deadband : Inport  Port=2
  Constant : Constant  Value=0  OutDataTypeStr=single
  Constant1 : Constant  Value=0  OutDataTypeStr=single
  Constant2 : Constant  OutDataTypeStr=single
  Constant3 : Constant  OutDataTypeStr=single
  remap_with_deadband : MATLAB Function  TreatAsAtomicUnit=on
  normalized_out : Outport
  wires:
  deadband/1 -> remap_with_deadband/6(deadband)
  Constant2/1 -> remap_with_deadband/5(out_max)
  Constant1/1 -> remap_with_deadband/4(out_min)
  Constant3/1 -> remap_with_deadband/3(in_max)
  Constant/1 -> remap_with_deadband/2(in_min)
  remap_with_deadband/1(norm_out) -> normalized_out/1
  raw_sbus_in/1 -> remap_with_deadband/1(raw_in)

== system torch_arm_telem/WAYPOINT CONTROLLER CMD/remap from min_spin to max ==
  raw_in : Inport
  Constant4 : Constant  Value=0  OutDataTypeStr=single
  Constant5 : Constant  Value=Aircraft.Control.motor_spin_min  OutDataTypeStr=single
  Constant6 : Constant  OutDataTypeStr=single
  Constant7 : Constant  OutDataTypeStr=single
  remap1 : MATLAB Function  TreatAsAtomicUnit=on
  norm_out : Outport
  wires:
  Constant6/1 -> remap1/5(out_max)
  Constant5/1 -> remap1/4(out_min)
  remap1/1(norm_out) -> norm_out/1
  Constant4/1 -> remap1/2(in_min)
  Constant7/1 -> remap1/3(in_max)
  raw_in/1 -> remap1/1(raw_in)

== system torch_arm_telem/cmd to raw pwm1/motor_PWM_denormalize ==
  normalized_input : Inport
  Constant : Constant  Value=0  OutDataTypeStr=single
  Constant1 : Constant  Value=1100  OutDataTypeStr=single
  Constant2 : Constant  Value=1950  OutDataTypeStr=single
  Constant3 : Constant  OutDataTypeStr=single
  remap : MATLAB Function  TreatAsAtomicUnit=on
  raw_output : Outport
  wires:
  Constant2/1 -> remap/5(out_max)
  Constant1/1 -> remap/4(out_min)
  Constant3/1 -> remap/3(in_max)
  Constant/1 -> remap/2(in_min)
  remap/1(raw_out) -> raw_output/1
  normalized_input/1 -> remap/1(norm_in)

== system torch_arm_telem/command selection/e_stop_norm ==
  raw_sbus_in : Inport
  Constant : Constant  Value=172  OutDataTypeStr=single
  Constant1 : Constant  Value=-1  OutDataTypeStr=single
  Constant2 : Constant  OutDataTypeStr=single
  Constant3 : Constant  Value=1811  OutDataTypeStr=single
  remap : MATLAB Function  TreatAsAtomicUnit=on
  normalized_out : Outport
  wires:
  Constant2/1 -> remap/5(out_max)
  Constant1/1 -> remap/4(out_min)
  Constant3/1 -> remap/3(in_max)
  Constant/1 -> remap/2(in_min)
  remap/1(norm_out) -> normalized_out/1
  raw_sbus_in/1 -> remap/1(raw_in)

== system torch_arm_telem/command selection/mode_norm ==
  raw_sbus_in : Inport
  Constant : Constant  Value=172  OutDataTypeStr=single
  Constant1 : Constant  Value=0  OutDataTypeStr=single
  Constant2 : Constant  Value=2  OutDataTypeStr=single
  Constant3 : Constant  Value=1811  OutDataTypeStr=single
  remap : MATLAB Function  TreatAsAtomicUnit=on
  normalized_out : Outport
  wires:
  raw_sbus_in/1 -> remap/1(raw_in)
  remap/1(norm_out) -> normalized_out/1
  Constant/1 -> remap/2(in_min)
  Constant3/1 -> remap/3(in_max)
  Constant1/1 -> remap/4(out_min)
  Constant2/1 -> remap/5(out_max)

== system torch_arm_telem/command selection/mode_norm1 ==
  raw_sbus_in : Inport
  Constant : Constant  Value=172  OutDataTypeStr=single
  Constant1 : Constant  Value=0  OutDataTypeStr=single
  Constant2 : Constant  OutDataTypeStr=single
  Constant3 : Constant  Value=1811  OutDataTypeStr=single
  remap : MATLAB Function  TreatAsAtomicUnit=on
  normalized_out : Outport
  wires:
  Constant2/1 -> remap/5(out_max)
  Constant1/1 -> remap/4(out_min)
  Constant3/1 -> remap/3(in_max)
  Constant/1 -> remap/2(in_min)
  remap/1(norm_out) -> normalized_out/1
  raw_sbus_in/1 -> remap/1(raw_in)

== system torch_arm_telem/command selection/pitch_norm_deadband ==
  raw_sbus_in : Inport
  deadband : Inport  Port=2
  Constant : Constant  Value=172  OutDataTypeStr=single
  Constant1 : Constant  Value=-1  OutDataTypeStr=single
  Constant2 : Constant  OutDataTypeStr=single
  Constant3 : Constant  Value=1811  OutDataTypeStr=single
  remap_with_deadband : MATLAB Function  TreatAsAtomicUnit=on
  normalized_out : Outport
  wires:
  deadband/1 -> remap_with_deadband/6(deadband)
  Constant2/1 -> remap_with_deadband/5(out_max)
  Constant1/1 -> remap_with_deadband/4(out_min)
  Constant3/1 -> remap_with_deadband/3(in_max)
  Constant/1 -> remap_with_deadband/2(in_min)
  remap_with_deadband/1(norm_out) -> normalized_out/1
  raw_sbus_in/1 -> remap_with_deadband/1(raw_in)

== system torch_arm_telem/command selection/roll_norm_deadband ==
  raw_sbus_in : Inport
  deadband : Inport  Port=2
  Constant : Constant  Value=172  OutDataTypeStr=single
  Constant1 : Constant  Value=-1  OutDataTypeStr=single
  Constant2 : Constant  OutDataTypeStr=single
  Constant3 : Constant  Value=1811  OutDataTypeStr=single
  remap_with_deadband : MATLAB Function  TreatAsAtomicUnit=on
  normalized_out : Outport
  wires:
  deadband/1 -> remap_with_deadband/6(deadband)
  Constant2/1 -> remap_with_deadband/5(out_max)
  Constant1/1 -> remap_with_deadband/4(out_min)
  Constant3/1 -> remap_with_deadband/3(in_max)
  Constant/1 -> remap_with_deadband/2(in_min)
  remap_with_deadband/1(norm_out) -> normalized_out/1
  raw_sbus_in/1 -> remap_with_deadband/1(raw_in)

== system torch_arm_telem/command selection/throttle_norm ==
  raw_sbus_in : Inport
  Constant : Constant  Value=172  OutDataTypeStr=single
  Constant1 : Constant  Value=0  OutDataTypeStr=single
  Constant2 : Constant  OutDataTypeStr=single
  Constant3 : Constant  Value=1811  OutDataTypeStr=single
  remap : MATLAB Function  TreatAsAtomicUnit=on
  normalized_out : Outport
  wires:
  raw_sbus_in/1 -> remap/1(raw_in)
  remap/1(norm_out) -> normalized_out/1
  Constant/1 -> remap/2(in_min)
  Constant3/1 -> remap/3(in_max)
  Constant1/1 -> remap/4(out_min)
  Constant2/1 -> remap/5(out_max)

== system torch_arm_telem/command selection/yaw_norm_deadband ==
  raw_sbus_in : Inport
  deadband : Inport  Port=2
  Constant : Constant  Value=172  OutDataTypeStr=single
  Constant1 : Constant  Value=-1  OutDataTypeStr=single
  Constant2 : Constant  OutDataTypeStr=single
  Constant3 : Constant  Value=1811  OutDataTypeStr=single
  remap_with_deadband : MATLAB Function  TreatAsAtomicUnit=on
  normalized_out : Outport
  wires:
  raw_sbus_in/1 -> remap_with_deadband/1(raw_in)
  remap_with_deadband/1(norm_out) -> normalized_out/1
  Constant/1 -> remap_with_deadband/2(in_min)
  Constant3/1 -> remap_with_deadband/3(in_max)
  Constant1/1 -> remap_with_deadband/4(out_min)
  Constant2/1 -> remap_with_deadband/5(out_max)
  deadband/1 -> remap_with_deadband/6(deadband)

== system torch_arm_telem/determine arm and mode selection/Failsafe_management ==
  note: - radio failsafe
  In Bus Element1 : Inport  PortName=inceptor  Element=failsafe
  manual_mode : Inport  Port=2
  motor_state : Inport  Port=3
  NOT : Logic  Operator=NOT  IconShape=distinctive  AllPortsSameDT=off  OutDataTypeStr=boolean
  Radio failsafe : Subsystem
  radio_failsafe_enabled : Outport
  wires:
  Radio failsafe/1(radio_failsafe_enabled) -> radio_failsafe_enabled/1
  manual_mode/1 -> Radio failsafe/2(manual_mode)
  motor_state/1 -> Radio failsafe/3(motor_state)
  In Bus Element1/1 -> NOT/1
  NOT/1 -> Radio failsafe/1(failsafe)

== system torch_arm_telem/determine arm and mode selection/Subsystem ==
  <e_stop> : Inport
  Abs1 : Abs  SaturateOnIntegerOverflow=off
  Compare To Constant : simulink/Logic and Bit Operations/Compare To Constant  relop=>=  const=0.98  OutDataTypeStr=boolean
  e_stop counter : Subsystem
  e_stop_filtered : Outport
  wires:
  Compare To Constant/1 -> e_stop counter/Enable
  Abs1/1 -> Compare To Constant/1
  <e_stop>/1 -> e_stop counter/1(motor_e_stop_raw), Abs1/1
  e_stop counter/1(e_stop_filtered) -> e_stop_filtered/1

== system torch_arm_telem/determine arm and mode selection/yaw_stick_arming ==
  note: yaw_stick arming
  <yaw> : Inport
  <throttle> : Inport  Port=2
  e_stop : Inport  Port=3
  AND : Logic  IconShape=distinctive  AllPortsSameDT=off  OutDataTypeStr=boolean
  Abs : Abs  SaturateOnIntegerOverflow=off
  Cast To Single : DataTypeConversion  OutDataTypeStr=single  SaturateOnIntegerOverflow=off  RndMeth=Floor
  Compare To Constant : simulink/Logic and Bit Operations/Compare To Constant  relop=>  const=0  OutDataTypeStr=boolean
  Compare To Constant1 : simulink/Logic and Bit Operations/Compare To Constant  relop=>=  const=0.95  OutDataTypeStr=boolean
  Compare To Constant2 : simulink/Logic and Bit Operations/Compare To Constant  relop=>=  const=3  OutDataTypeStr=boolean
  Compare To Constant3 : simulink/Logic and Bit Operations/Compare To Constant  relop=<=  const=0.03  OutDataTypeStr=boolean
  Compare To Constant4 : simulink/Logic and Bit Operations/Compare To Constant  relop=>=  const=0.5  OutDataTypeStr=boolean
  Constant : Constant  Value=0  OutDataTypeStr=boolean  LockScale=on
  Enabled Subsystem : Subsystem  TreatAsAtomicUnit=on
  OR : Logic  Operator=OR  IconShape=distinctive  AllPortsSameDT=off  OutDataTypeStr=boolean
  Sum : Sum  Inputs=-+|
  Switch : Switch  Criteria=u2 > Threshold  SaturateOnIntegerOverflow=off  InputSameDT=off
  Unit Delay : UnitDelay  SampleTime=-1  HasFrameUpgradeWarning=on
  manual_arming : Subsystem
  arm_state : Outport
  wires:
  Enabled Subsystem/1(time_arm_valid_s) -> Compare To Constant2/1
  Abs/1 -> Compare To Constant1/1
  Compare To Constant1/1 -> AND/2, Enabled Subsystem/1(yaw_input)
  Compare To Constant4/1 -> manual_arming/1(yaw_arm)
  AND/1 -> Enabled Subsystem/Enable
  <yaw>/1 -> Compare To Constant4/1, Abs/1
  <throttle>/1 -> Compare To Constant3/1
  Compare To Constant3/1 -> AND/1
  Constant/1 -> Switch/1
  manual_arming/1(arm_state) -> Switch/3
  Switch/1 -> arm_state/1
  e_stop/1 -> OR/1, Switch/2
  OR/1 -> manual_arming/Trigger
  Compare To Constant2/1 -> Cast To Single/1
  Sum/1 -> Compare To Constant/1
  Unit Delay/1 -> Sum/1
  Cast To Single/1 -> Unit Delay/1, Sum/2
  Compare To Constant/1 -> OR/2

== system torch_arm_telem/ANGLE CONTROLLER1/Pitch Controller/pitch_D_DLPF ==
  raw_val : Inport
  freq_cut : Inport  Port=2
  Constant : Constant  Value=frameRate_hz  OutDataTypeStr=single
  MATLAB Function : MATLAB Function  TreatAsAtomicUnit=on
  Unit Delay : UnitDelay  SampleTime=-1  HasFrameUpgradeWarning=on
  filtered_val : Outport
  wires:
  freq_cut/1 -> MATLAB Function/3(freq_cut)
  MATLAB Function/1(filtered_val) -> Unit Delay/1, filtered_val/1
  Unit Delay/1 -> MATLAB Function/1(prev_val)
  raw_val/1 -> MATLAB Function/2(raw_val)
  Constant/1 -> MATLAB Function/4(samp_freq)

== system torch_arm_telem/ANGLE CONTROLLER1/Pitch Controller/pitch_input_DLPF ==
  raw_val : Inport
  freq_cut : Inport  Port=2
  Constant : Constant  Value=frameRate_hz  OutDataTypeStr=single
  MATLAB Function : MATLAB Function  TreatAsAtomicUnit=on
  Unit Delay : UnitDelay  SampleTime=-1  HasFrameUpgradeWarning=on
  filtered_val : Outport
  wires:
  Constant/1 -> MATLAB Function/4(samp_freq)
  raw_val/1 -> MATLAB Function/2(raw_val)
  Unit Delay/1 -> MATLAB Function/1(prev_val)
  MATLAB Function/1(filtered_val) -> filtered_val/1, Unit Delay/1
  freq_cut/1 -> MATLAB Function/3(freq_cut)

== system torch_arm_telem/ANGLE CONTROLLER1/Roll Controller/roll_D_DLPF ==
  raw_val : Inport
  freq_cut : Inport  Port=2
  Constant : Constant  Value=frameRate_hz  OutDataTypeStr=single
  MATLAB Function : MATLAB Function  TreatAsAtomicUnit=on
  Unit Delay : UnitDelay  SampleTime=-1  HasFrameUpgradeWarning=on
  filtered_val : Outport
  wires:
  freq_cut/1 -> MATLAB Function/3(freq_cut)
  MATLAB Function/1(filtered_val) -> Unit Delay/1, filtered_val/1
  Unit Delay/1 -> MATLAB Function/1(prev_val)
  raw_val/1 -> MATLAB Function/2(raw_val)
  Constant/1 -> MATLAB Function/4(samp_freq)

== system torch_arm_telem/ANGLE CONTROLLER1/Yaw Rate Controller/heading_error ==
  heading_cmd_rad : Inport
  heading_rad : Inport  Port=2
  Abs : Abs  SaturateOnIntegerOverflow=off
  Compare To Constant : simulink/Logic and Bit Operations/Compare To Constant  relop=>  const=pi  OutDataTypeStr=boolean
  Constant : Constant  Value=2*pi  OutDataTypeStr=single
  Product : Product
  Sign : Signum
  Subtract : Sum  Inputs=+-
  Subtract1 : Sum  Inputs=+-
  Switch : Switch  Criteria=u2 > Threshold  SaturateOnIntegerOverflow=off  InputSameDT=off
  heading_error_rad : Outport
  wires:
  heading_cmd_rad/1 -> Subtract/1
  heading_rad/1 -> Subtract/2
  Subtract/1 -> Abs/1, Switch/3, Subtract1/1, Sign/1
  Compare To Constant/1 -> Switch/2
  Subtract1/1 -> Switch/1
  Switch/1 -> heading_error_rad/1
  Abs/1 -> Compare To Constant/1
  Sign/1 -> Product/1
  Product/1 -> Subtract1/2
  Constant/1 -> Product/2

== system torch_arm_telem/ANGLE CONTROLLER1/Yaw Rate Controller/set_tar_heading when heading_rate_cmd == 0 ==
  heading_rad : Inport
  Enable : EnablePort
  target_heading_rad : Outport
  wires:
  heading_rad/1 -> target_heading_rad/1

== system torch_arm_telem/ANGLE CONTROLLER1/Yaw Rate Controller/yaw_D_DLPF ==
  raw_val : Inport
  freq_cut : Inport  Port=2
  Constant : Constant  Value=frameRate_hz  OutDataTypeStr=single
  MATLAB Function : MATLAB Function  TreatAsAtomicUnit=on
  Unit Delay : UnitDelay  SampleTime=-1  HasFrameUpgradeWarning=on
  filtered_val : Outport
  wires:
  freq_cut/1 -> MATLAB Function/3(freq_cut)
  MATLAB Function/1(filtered_val) -> Unit Delay/1, filtered_val/1
  Unit Delay/1 -> MATLAB Function/1(prev_val)
  raw_val/1 -> MATLAB Function/2(raw_val)
  Constant/1 -> MATLAB Function/4(samp_freq)

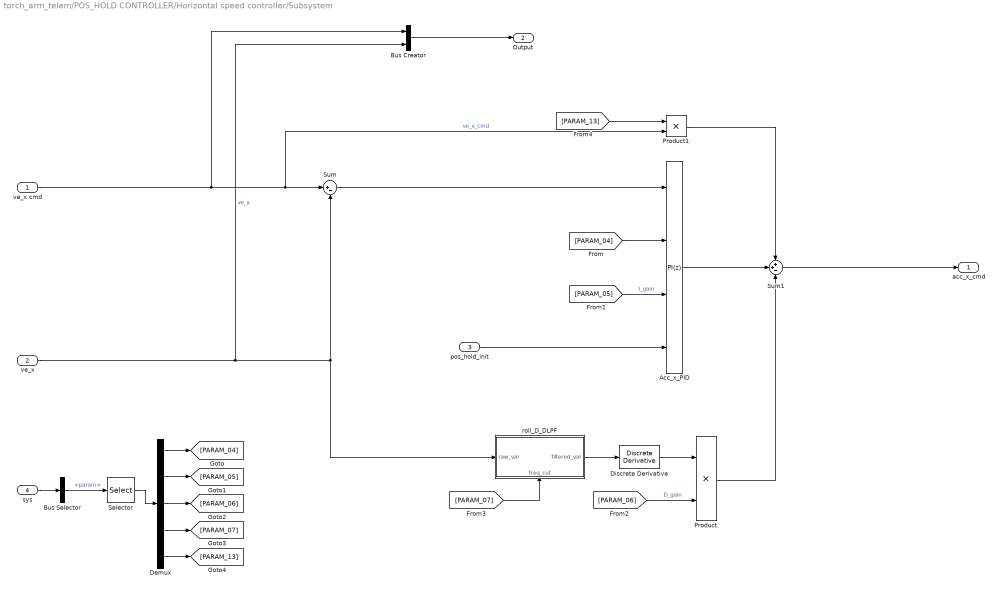
== system torch_arm_telem/POS_HOLD CONTROLLER/Horizontal speed controller/Subsystem ==
  ve_x cmd : Inport
  ve_x : Inport  Port=2
  pos_hold_init : Inport  Port=3
  sys : Inport  Port=4
  Acc_x_PID : slpidlib/PID Controller  Controller=PI  Form=Parallel  TimeDomain=Discrete-time  UseExternalTs=off  SampleTime=framePeriod_s  IntegratorMethod=Forward Euler  FilterMethod=Forward Euler  ControllerParametersSource=external  P=0.335  I=0.005  UseKiTs=off  D=0  UseExternalDerivativeSource=off  N=100  UseFilter=off  TunerSelectOption=Transfer Function Based (PID Tuner App)  InitialConditionSource=internal  InitialConditionForIntegrator=0  InitialConditionForFilter=0  DifferentiatorICPrevScaledInput=0  ExternalReset=either  TrackingMode=off  Kt=1  LimitOutput=off  SatLimitsSource=internal  UpperSaturationLimit=Aircraft.Control.pitch_angle_lim  LowerSaturationLimit=-Aircraft.Control.pitch_angle_lim  LinearizeAsGain=off  AntiWindupMode=clamping  Kb=1  LimitIntegrator=off  UpperIntegratorSaturationLimit=inf  LowerIntegratorSaturationLimit=-inf  POutMin=[]  POutMax=[]  IOutMin=[]  IOutMax=[]  DOutMin=[]  DOutMax=[]  NOutMin=[]  NOutMax=[]  SumOutMin=[]  SumOutMax=[]  SaturationOutMin=[]  SaturationOutMax=[]  PParamMin=[]  PParamMax=[]  IParamMin=[]  IParamMax=[]  DParamMin=[]  DParamMax=[]  NParamMin=[]  NParamMax=[]  KbParamMin=[]  KbParamMax=[]  KtParamMin=[]  KtParamMax=[]  KbOutMin=[]  KbOutMax=[]  KtOutMin=[]  KtOutMax=[]  IntegratorOutMin=[]  IntegratorOutMax=[]  FilterOutMin=[]  FilterOutMax=[]  SumI1OutMin=[]  SumI1OutMax=[]  SumI2OutMin=[]  SumI2OutMax=[]  SumI3OutMin=[]  SumI3OutMax=[]  SumI4OutMin=[]  SumI4OutMax=[]  SumDOutMin=[]  SumDOutMax=[]  DifferentiatorOutMin=[]  DifferentiatorOutMax=[]  FilterDiffOutCoefMin=[]  FilterDiffOutCoefMax=[]  ReciprocalOutMin=[]  ReciprocalOutMax=[]  SumDenOutMin=[]  SumDenOutMax=[]  SumNumOutMin=[]  SumNumOutMax=[]  DivideOutMin=[]  DivideOutMax=[]  UdiffTsProdOutMin=[]  UdiffTsProdOutMax=[]  NTsProdOutMin=[]  NTsProdOutMax=[]  UintegralTsProdOutMin=[]  UintegralTsProdOutMax=[]  UngainTsProdOutMin=[]  UngainTsProdOutMax=[]  ClampingZeroOutDataTypeStr=Inherit: Inherit via back propagation  ClampingZeroOutMin=[]  ClampingZeroOutMax=[]  FilterDenConstantOutDataTypeStr=Inherit: Inherit via back propagation  FilterDenConstantOutMin=[]  FilterDenConstantOutMax=[]  PCopyOutDataTypeStr=Inherit: Inherit via back propagation  PCopyOutMin=[]  PCopyOutMax=[]  NCopyOutDataTypeStr=Inherit: Inherit via back propagation  NCopyOutMin=[]  NCopyOutMax=[]  IntegratorContinuousStateAttributes=''  IntegratorStateMustResolveToSignalObject=off  IntegratorRTWStateStorageClass=Auto  FilterContinuousStateAttributes=''  FilterStateMustResolveToSignalObject=off  FilterRTWStateStorageClass=Auto  ParallelPVariant=ExternalParameters  IdealPVariant=Disabled  IVariant=ExternalParameters  DVariant=Disabled  IntegratorVariant=Discrete  SatVariant=Disabled  AWVariant=Passthrough  PCopyVariant=Disabled  TRVariant=Disabled  FdbkBlocksVariant=Forward  IdealPFdbkVariant=Disabled  SatFdbkVariant=Disabled  DerivativeFilterVariant=Disabled  NVariant=Disabled  NCopyVariant=Disabled_SignalSpec  FilterICVariant=Disabled  IntegratorICVariant=InternalICs  ExternalResetVariant=ExternalReset  TRSumVariant=Passthrough  SumFdbkVariant=Disabled  SumVariant=Sum_PI  TsampFilterVariant=InternalTs  TsampNgainVariant=Passthrough  TsampIntegralVariant=Disabled_SignalSpec  ExternalSaturationOutDataTypeStr=Inherit: Same as second input  DerivativeSourceVariant=Disabled
  Bus Creator : BusCreator  Inputs=2
  Bus Selector : BusSelector  OutputSignals=Telemetry Data.param
  Demux : Demux  Outputs=5
  Discrete Derivative : simulink/Discrete/Discrete Derivative  gainval=1.0  ICPrevScaledInput=0.0  OutMin=[]  OutMax=[]  OutDataType=fixdt(1, 16)  OutScaling=2^-10  DoSatur=off
  Product : Product
  Product1 : Product
  Selector : Selector  IndexMode=Zero-based  InputPortWidth=24  IndexOptions=Index vector (dialog)  Indices=[4 5 6 7 13]  OutputSizes=1
  Sum : Sum  Inputs=|+-
  Sum1 : Sum  Inputs=++-
  roll_D_DLPF : Subsystem
      settings: PortSchema="{\"entries\":[{\"content\":{\"sides\":[{\"content\":{\"connectorIds\":[\"In1\"]},\"type\":\"ConnectorPlacement.EquallySpacedRectSide\",\"uuid\":\"20236834-aeb3-4c5b-bb2e-f84447e752b5\"},{\"content\":{\"connectorIds\":[\"Out1\"],\"side\":\"RIGHT\"},\"type\":\"ConnectorPlacement.EquallySpacedRectSide\",\"uuid\":\"d668f9a1-a3df-4207-8bf1-99fb838e59b2\"},{\"content\":{\"connectorIds\":[],\"side\":\"TOP\"},\"type\":\"ConnectorPlacement.EquallySpacedRectSide\",\"uuid\":\"66cceb06-f4bc-4278-b965-2427292e46df\"},{\"content\":{\"connectorIds\":[\"In2\"],\"side\":\"BOTTOM\"},\"type\":\"ConnectorPlacement.EquallySpacedRectSide\",\"uuid\":\"8fdaac6a-cb03-4bd4-87bb-7bafd10bc297\"}]},\"type\":\"ConnectorPlacement.EquallySpacedConnector\",\"uuid\":\"3dc29a9a-e794-478d-b7df-452e6c2d3f66\"}],\"packageUris\":[\"http://schema.mathworks.com/mf0/Connector/R2020b\"],\"version\":\"1.0\"}"
  acc_x_cmd : Outport
  Output : Outport  Port=2
  wires:
  ve_x/1 -> Bus Creator/2, roll_D_DLPF/1(raw_val), Sum/2  "ve_x"
  Sum/1 -> Acc_x_PID/1
  [PARAM_04] -> Acc_x_PID/2
  [PARAM_05] -> Acc_x_PID/3  "I_gain"
  pos_hold_init/1 -> Acc_x_PID/4
  [PARAM_06] -> Product/2  "D_gain"
  Discrete Derivative/1 -> Product/1
  [PARAM_07] -> roll_D_DLPF/2(freq_cut)
  roll_D_DLPF/1(filtered_val) -> Discrete Derivative/1
  Bus Creator/1 -> Output/1
  ve_x cmd/1 -> Product1/2, Sum/1, Bus Creator/1  "ve_x_cmd"
  Sum1/1 -> acc_x_cmd/1
  sys/1 -> Bus Selector/1
  Bus Selector/1 -> Selector/1  "<param>"
  Selector/1 -> Demux/1
  Demux/1 -> [PARAM_04]
  Demux/3 -> [PARAM_06]
  Demux/2 -> [PARAM_05]
  Demux/4 -> [PARAM_07]
  Demux/5 -> [PARAM_13]
  [PARAM_13] -> Product1/1
  Product1/1 -> Sum1/1
  Acc_x_PID/1 -> Sum1/2
  Product/1 -> Sum1/3
